simulink model "sbic_proj_olderVersion"  (R2020a)
settings: Solver=VariableStepAuto  StartTime=0.0  StopTime=200  RelTol=1e-3
libraries: fuzblock x6
settings Model: Creator=tecas  LastModifiedBy=joaoc

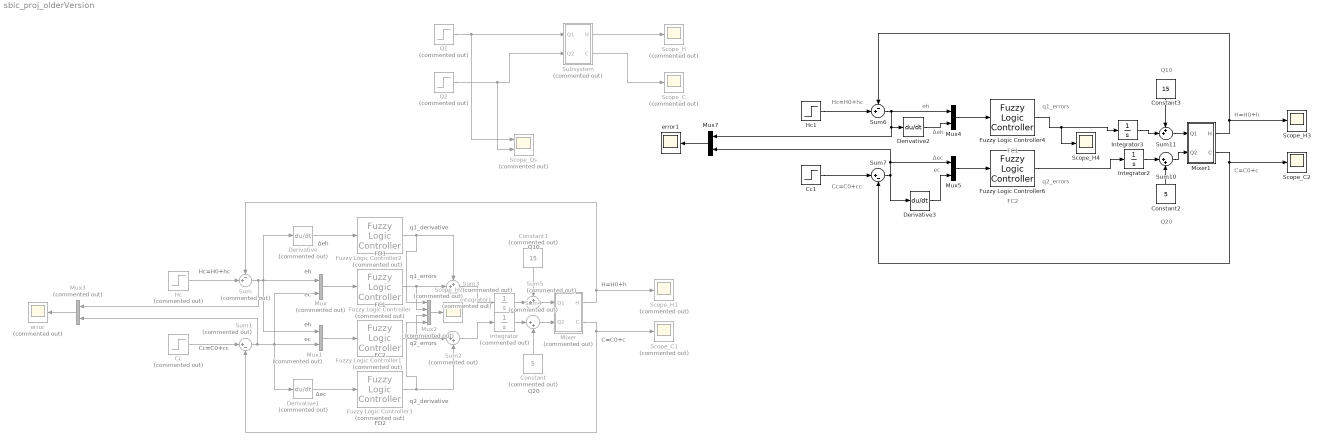
== system sbic_proj_olderVersion ==
  note: Hc=H0+hc
  note: eh
  note: FC1
  note: Q20
  note: q1_errors
  note: q2_errors
  note: Q10
  note: FC2
  note: FD2
  note: FD1
  note: eh
  note: Δeh
  note: Δec
  note: ec
  note: ec
  note: Cc=C0+cc
  note: H=H0+h
  note: C=C0+c
  note: q2_derivative
  note: q1_derivative
  note: Δeh
  note: Δec
  note: Cc=C0+cc
  note: ec
  note: Hc=H0+hc
  note: eh
  note: FC1
  note: Q20
  note: q1_errors
  note: q2_errors
  note: Q10
  note: C=C0+c
  note: H=H0+h
  note: FC2
  Cc : Step  Commented=on  Time=15  Before=5  After=5  SampleTime=0
  Cc1 : Step  Time=15  After=5  SampleTime=0
  Constant : Constant  Commented=on  Value=5
  Constant1 : Constant  Commented=on  Value=15
  Constant2 : Constant  Value=5
  Constant3 : Constant  Value=15
  Derivative : Derivative  Commented=on
  Derivative1 : Derivative  Commented=on
  Derivative2 : Derivative
  Derivative3 : Derivative
  Fuzzy Logic Controller : fuzblock/Fuzzy Logic  Controller  Commented=on  FIS=FC3  OutputSampleNumber=101  DataType=double  FuzzifiedInputs=off  RuleFiringStrengths=off  RuleOutputs=off  AggregatedOutputs=off  SimulateUsing=Interpreted execution  OutOfRangeInputValueMessage=warning  NoRuleFiredMessage=warning  EmptyOutputFuzzySetMessage=warning
  Fuzzy Logic Controller1 : fuzblock/Fuzzy Logic  Controller  Commented=on  FIS=FC2  OutputSampleNumber=101  DataType=double  FuzzifiedInputs=off  RuleFiringStrengths=off  RuleOutputs=off  AggregatedOutputs=off  SimulateUsing=Interpreted execution  OutOfRangeInputValueMessage=warning  NoRuleFiredMessage=warning  EmptyOutputFuzzySetMessage=warning
  Fuzzy Logic Controller2 : fuzblock/Fuzzy Logic  Controller  Commented=on  FIS=FD  OutputSampleNumber=101  DataType=double  FuzzifiedInputs=off  RuleFiringStrengths=off  RuleOutputs=off  AggregatedOutputs=off  SimulateUsing=Interpreted execution  OutOfRangeInputValueMessage=warning  NoRuleFiredMessage=warning  EmptyOutputFuzzySetMessage=warning
  Fuzzy Logic Controller3 : fuzblock/Fuzzy Logic  Controller  Commented=on  FIS=FD  OutputSampleNumber=101  DataType=double  FuzzifiedInputs=off  RuleFiringStrengths=off  RuleOutputs=off  AggregatedOutputs=off  SimulateUsing=Interpreted execution  OutOfRangeInputValueMessage=warning  NoRuleFiredMessage=warning  EmptyOutputFuzzySetMessage=warning
  Fuzzy Logic Controller4 : fuzblock/Fuzzy Logic  Controller  FIS=FC1_ex3  OutputSampleNumber=101  DataType=double  FuzzifiedInputs=off  RuleFiringStrengths=off  RuleOutputs=off  AggregatedOutputs=off  SimulateUsing=Interpreted execution  OutOfRangeInputValueMessage=warning  NoRuleFiredMessage=warning  EmptyOutputFuzzySetMessage=warning
  Fuzzy Logic Controller6 : fuzblock/Fuzzy Logic  Controller  FIS=FC2_ex3  OutputSampleNumber=101  DataType=double  FuzzifiedInputs=off  RuleFiringStrengths=off  RuleOutputs=off  AggregatedOutputs=off  SimulateUsing=Interpreted execution  OutOfRangeInputValueMessage=warning  NoRuleFiredMessage=warning  EmptyOutputFuzzySetMessage=warning
  Hc : Step  Commented=on  Time=15  Before=5  After=5  SampleTime=0
  Hc1 : Step  Time=25  After=5  SampleTime=0
  Integrator : Integrator  Commented=on
  Integrator1 : Integrator  Commented=on
  Integrator2 : Integrator
  Integrator3 : Integrator
  Mixer : Subsystem  Commented=on
  Mixer1 : Subsystem
  Mux : Mux  Commented=on  Inputs=2
  Mux1 : Mux  Commented=on  Inputs=2
  Mux2 : Mux  Commented=on
  Mux3 : Mux  Commented=on  Inputs=2
  Mux4 : Mux  Inputs=2
  Mux5 : Mux  Inputs=2
  Mux7 : Mux  Inputs=2
  Q1 : Step  Commented=on  Time=15  Before=15  After=15  SampleTime=0
  Q2 : Step  Commented=on  Time=15  Before=5  After=5  SampleTime=0
  Scope_C : Scope  Commented=on
  Scope_C1 : Scope  Commented=on
  Scope_C2 : Scope
  Scope_H : Scope  Commented=on
  Scope_H1 : Scope  Commented=on
  Scope_H2 : Scope  Commented=on
  Scope_H3 : Scope
  Scope_H4 : Scope
  Scope_Qs : Scope  Commented=on  NumInputPorts=2
  Subsystem : Subsystem  Commented=on
  Sum : Sum  Commented=on  Inputs=-+|
  Sum1 : Sum  Commented=on  Inputs=|+-
  Sum10 : Sum  Inputs=|++
  Sum11 : Sum  Inputs=++|
  Sum2 : Sum  Commented=on  Inputs=|++
  Sum3 : Sum  Commented=on  Inputs=++|
  Sum4 : Sum  Commented=on  Inputs=|++
  Sum5 : Sum  Commented=on  Inputs=++|
  Sum6 : Sum  Inputs=-+|
  Sum7 : Sum  Inputs=|+-
  error : Scope  Commented=on
  error1 : Scope
  wires:
  Q1/1 -> Subsystem/1(Q1), Scope_Qs/1
  Q2/1 -> Scope_Qs/2, Subsystem/2(Q2)
  Subsystem/1(H) -> Scope_H/1
  Subsystem/2(C) -> Scope_C/1
  Mixer/2(C) -> Scope_C1/1, Sum1/2
  Mixer/1(H) -> Sum/1, Scope_H1/1
  Mux/1 -> Fuzzy Logic Controller/1
  Mux1/1 -> Fuzzy Logic Controller1/1
  Hc/1 -> Sum/2
  Cc/1 -> Sum1/1
  Sum1/1 -> Mux3/2, Mux/2, Mux1/2, Derivative1/1
  Fuzzy Logic Controller1/1 -> Mux2/3, Sum2/1
  Sum2/1 -> Integrator/1
  Fuzzy Logic Controller/1 -> Mux2/2, Sum3/2
  Sum3/1 -> Integrator1/1
  Integrator/1 -> Sum4/1
  Sum4/1 -> Mixer/2(Q2)
  Integrator1/1 -> Sum5/2
  Sum5/1 -> Mixer/1(Q1)
  Constant/1 -> Sum4/2
  Constant1/1 -> Sum5/1
  Derivative1/1 -> Fuzzy Logic Controller3/1
  Derivative/1 -> Fuzzy Logic Controller2/1
  Fuzzy Logic Controller2/1 -> Mux2/1, Sum3/1
  Fuzzy Logic Controller3/1 -> Mux2/4, Sum2/2
  Mux2/1 -> Scope_H2/1
  Mux3/1 -> error/1
  Sum/1 -> Mux3/1, Mux1/1, Mux/1, Derivative/1
  Sum6/1 -> Mux4/1, Mux7/1, Derivative2/1
  Sum7/1 -> Mux5/1, Mux7/2, Derivative3/1
  Fuzzy Logic Controller4/1 -> Scope_H4/1, Integrator3/1
  Hc1/1 -> Sum6/2
  Sum11/1 -> Mixer1/1(Q1)
  Integrator3/1 -> Sum11/2
  Integrator2/1 -> Sum10/1
  Constant3/1 -> Sum11/1
  Mux7/1 -> error1/1
  Cc1/1 -> Sum7/1
  Derivative3/1 -> Mux5/2
  Mixer1/1(H) -> Sum6/1, Scope_H3/1
  Mux4/1 -> Fuzzy Logic Controller4/1
  Mux5/1 -> Fuzzy Logic Controller6/1
  Mixer1/2(C) -> Scope_C2/1, Sum7/2
  Derivative2/1 -> Mux4/2
  Fuzzy Logic Controller6/1 -> Integrator2/1
  Constant2/1 -> Sum10/2
  Sum10/1 -> Mixer1/2(Q2)

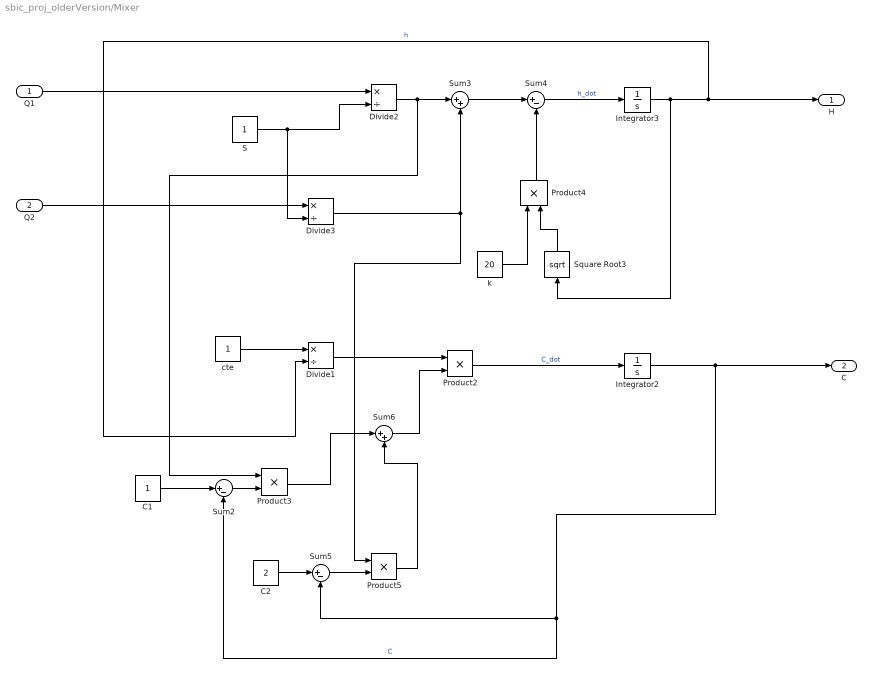
== system sbic_proj_olderVersion/Mixer ==
  Q1 : Inport
  Q2 : Inport  Port=2
  C1 : Constant
  C2 : Constant  Value=2
  Divide1 : Product  Inputs=*/
  Divide2 : Product  Inputs=*/
  Divide3 : Product  Inputs=*/
  Integrator2 : Integrator  InitialCondition=1.25
  Integrator3 : Integrator  InitialCondition=1
  Product{2..5} (4 alike) : Product
  S : Constant
  Square Root3 : Sqrt  SaturateOnIntegerOverflow=on
  Sum2 : Sum  Inputs=|+-
  Sum3 : Sum  Inputs=|++
  Sum4 : Sum  Inputs=|+-
  Sum5 : Sum  Inputs=|+-
  Sum6 : Sum  Inputs=|++
  cte : Constant
  k : Constant  Value=20
  H : Outport
  C : Outport  Port=2
  wires:
  C1/1 -> Sum2/1
  C2/1 -> Sum5/1
  Product4/1 -> Sum4/2
  Product2/1 -> Integrator2/1  "C_dot"
  Integrator2/1 -> C/1, Sum5/2, Sum2/2  "C"
  S/1 -> Divide2/2, Divide3/2
  Integrator3/1 -> H/1, Divide1/2, Square Root3/1  "h"
  Sum3/1 -> Sum4/1
  Sum2/1 -> Product3/2
  Product5/1 -> Sum6/2
  Product3/1 -> Sum6/1
  Divide3/1 -> Product5/1, Sum3/2
  Sum5/1 -> Product5/2
  Sum4/1 -> Integrator3/1  "h_dot"
  cte/1 -> Divide1/1
  Divide2/1 -> Product3/1, Sum3/1
  Square Root3/1 -> Product4/2
  Q2/1 -> Divide3/1
  Q1/1 -> Divide2/1
  Divide1/1 -> Product2/1
  Sum6/1 -> Product2/2
  k/1 -> Product4/1

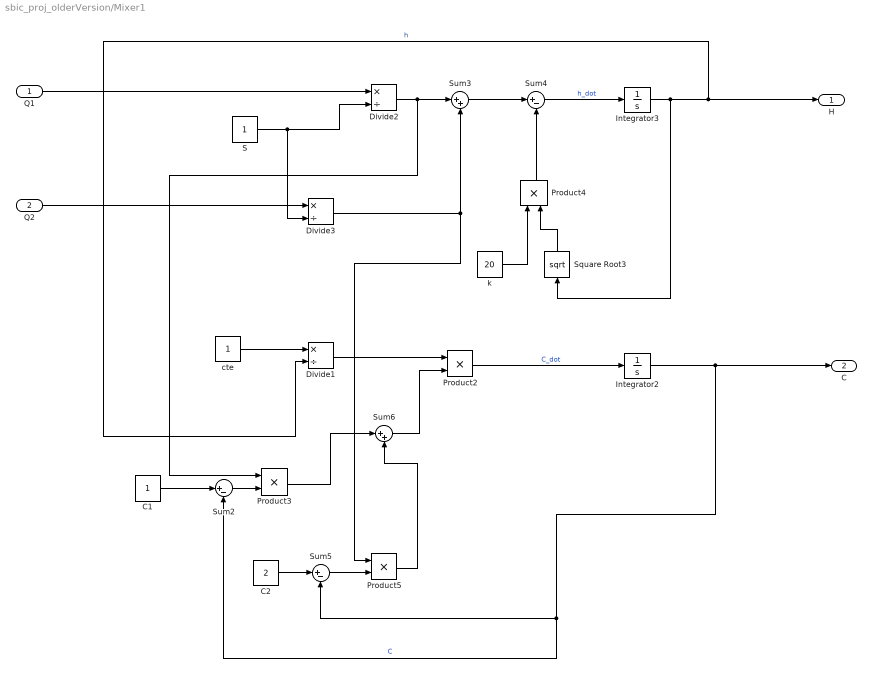
== system sbic_proj_olderVersion/Mixer1 ==
  Q1 : Inport
  Q2 : Inport  Port=2
  C1 : Constant
  C2 : Constant  Value=2
  Divide1 : Product  Inputs=*/
  Divide2 : Product  Inputs=*/
  Divide3 : Product  Inputs=*/
  Integrator2 : Integrator  InitialCondition=1.25
  Integrator3 : Integrator  InitialCondition=1
  Product{2..5} (4 alike) : Product
  S : Constant
  Square Root3 : Sqrt  SaturateOnIntegerOverflow=on
  Sum2 : Sum  Inputs=|+-
  Sum3 : Sum  Inputs=|++
  Sum4 : Sum  Inputs=|+-
  Sum5 : Sum  Inputs=|+-
  Sum6 : Sum  Inputs=|++
  cte : Constant
  k : Constant  Value=20
  H : Outport
  C : Outport  Port=2
  wires:
  C1/1 -> Sum2/1
  C2/1 -> Sum5/1
  Product4/1 -> Sum4/2
  Product2/1 -> Integrator2/1  "C_dot"
  Integrator2/1 -> C/1, Sum5/2, Sum2/2  "C"
  S/1 -> Divide2/2, Divide3/2
  Integrator3/1 -> H/1, Divide1/2, Square Root3/1  "h"
  Sum3/1 -> Sum4/1
  Sum2/1 -> Product3/2
  Product5/1 -> Sum6/2
  Product3/1 -> Sum6/1
  Divide3/1 -> Product5/1, Sum3/2
  Sum5/1 -> Product5/2
  Sum4/1 -> Integrator3/1  "h_dot"
  cte/1 -> Divide1/1
  Divide2/1 -> Product3/1, Sum3/1
  Square Root3/1 -> Product4/2
  Q2/1 -> Divide3/1
  Q1/1 -> Divide2/1
  Divide1/1 -> Product2/1
  Sum6/1 -> Product2/2
  k/1 -> Product4/1

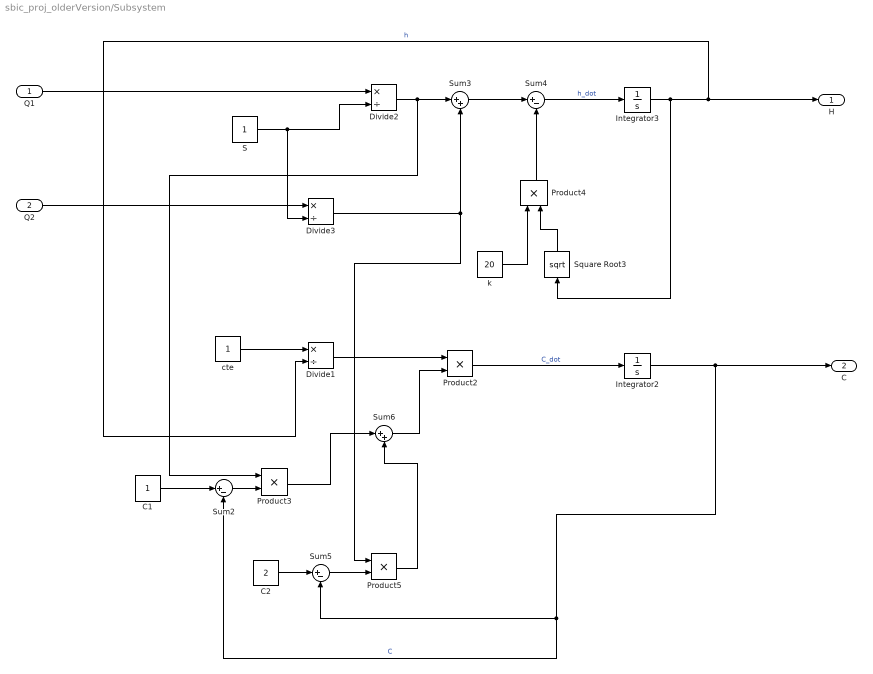
== system sbic_proj_olderVersion/Subsystem ==
  Q1 : Inport
  Q2 : Inport  Port=2
  C1 : Constant
  C2 : Constant  Value=2
  Divide1 : Product  Inputs=*/
  Divide2 : Product  Inputs=*/
  Divide3 : Product  Inputs=*/
  Integrator2 : Integrator  InitialCondition=1.25
  Integrator3 : Integrator  InitialCondition=1
  Product{2..5} (4 alike) : Product
  S : Constant
  Square Root3 : Sqrt  SaturateOnIntegerOverflow=on
  Sum2 : Sum  Inputs=|+-
  Sum3 : Sum  Inputs=|++
  Sum4 : Sum  Inputs=|+-
  Sum5 : Sum  Inputs=|+-
  Sum6 : Sum  Inputs=|++
  cte : Constant
  k : Constant  Value=20
  H : Outport
  C : Outport  Port=2
  wires:
  C1/1 -> Sum2/1
  C2/1 -> Sum5/1
  Product4/1 -> Sum4/2
  Product2/1 -> Integrator2/1  "C_dot"
  Integrator2/1 -> C/1, Sum5/2, Sum2/2  "C"
  S/1 -> Divide2/2, Divide3/2
  Integrator3/1 -> H/1, Divide1/2, Square Root3/1  "h"
  Sum3/1 -> Sum4/1
  Sum2/1 -> Product3/2
  Product5/1 -> Sum6/2
  Product3/1 -> Sum6/1
  Divide3/1 -> Product5/1, Sum3/2
  Sum5/1 -> Product5/2
  Sum4/1 -> Integrator3/1  "h_dot"
  cte/1 -> Divide1/1
  Divide2/1 -> Product3/1, Sum3/1
  Square Root3/1 -> Product4/2
  Q2/1 -> Divide3/1
  Q1/1 -> Divide2/1
  Divide1/1 -> Product2/1
  Sum6/1 -> Product2/2
  k/1 -> Product4/1
